simulink library "AuxEq_Lib"  (Simulink 8.0)
settings: Solver=ode45  SolverMode=SingleTasking  StartTime=0.0  StopTime=10.0  RelTol=1e-3
values from neighbouring files (symbols this model uses):
  TrimCondition =     [UAV_trimcondition.mat]
libraries: aerolibasang x3, Navigation_Lib x1, simulink x1
settings Model: Creator=Paul Freeman  LastModifiedBy=brtaylor

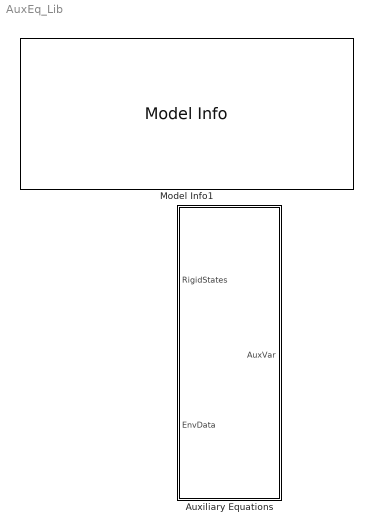
== system AuxEq_Lib ==
  Auxiliary Equations : Subsystem
  Model Info1 : simulink/Model-Wide Utilities/Model Info  InitialBlockCM=None  BlockCM=None  Frame=on  DisplayStringWithTags=|  HorizontalTextAlignment=Left  LeftAlignmentValue=0.02  SourceBlockDiagram=AuxEq_Lib  TagMaxNumber=20
      | MODEL INFORMATION
      | Auxiliary Equations Library
      | 
      | University of Minnesota
      | Aerospace Engineering and Mechanics
      | Copyright 2011 Regents of the University of Minnesota. All rights reserved.
      | 
      | == SVN Info ==
      | Last modified by %<LastModifiedBy> on %<LastModificationDate>

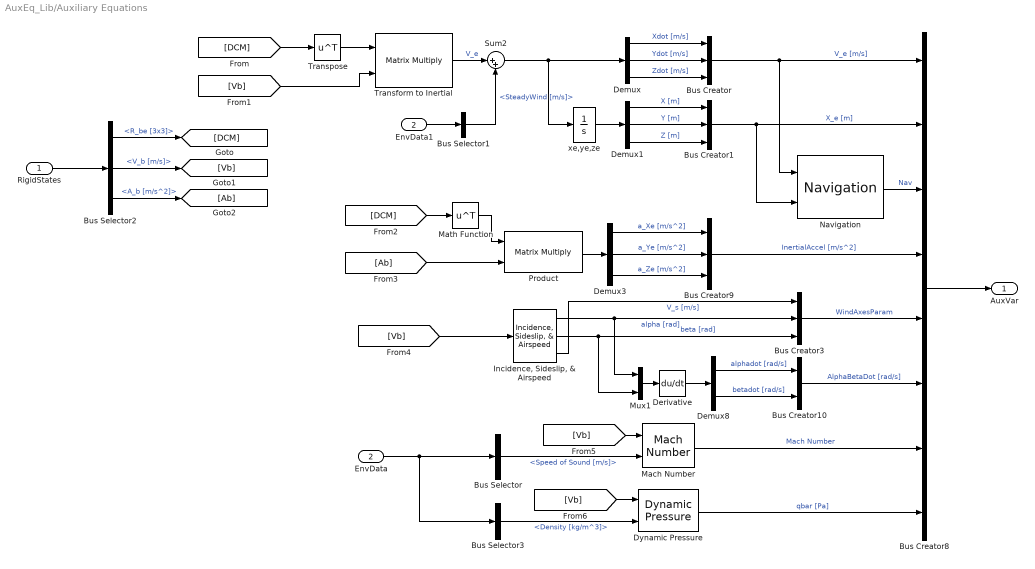
== system AuxEq_Lib/Auxiliary Equations ==
  RigidStates : Inport
  EnvData : Inport  Port=2
  Bus Creator{,1,3,9} (4 alike) : BusCreator  Inputs=3
  Bus Creator10 : BusCreator  Inputs=2
  Bus Creator8 : BusCreator  Inputs=8
  Bus Selector : BusSelector  OutputSignals=Speed of Sound [m/s]
  Bus Selector1 : BusSelector  OutputSignals=SteadyWind [m/s]
  Bus Selector2 : BusSelector  OutputSignals=R_be [3x3],V_b [m/s],A_b [m/s^2]
  Bus Selector3 : BusSelector  OutputSignals=Density [kg/m^3]
  Demux : Demux  Outputs=3
  Demux1 : Demux  Outputs=3
  Demux3 : Demux  Outputs=3
  Demux8 : Demux  Outputs=2
  Derivative : Derivative
  Dynamic Pressure : aerolibasang/Dynamic Pressure
  EnvData1 : InportShadow  Port=2
  "Incidence, Sideslip, & Airspeed" : aerolibasang/Incidence, Sideslip, & Airspeed
  Mach Number : aerolibasang/Mach Number
  Math Function : Math  Operator=transpose  SaturateOnIntegerOverflow=on
  Mux1 : Mux  Inputs=2
  Navigation : Navigation_Lib/Navigation  Description=|
      | This model produces the followng navigation data for the UAV flight:
      |                                                                     
      | * Geodetic Latitude                                                 
      | * Geodetic Longitude                                                
      | * Geodetic Altitude                                                 
      | * Altitude above Mean Sea Level                                     
      | * Gravitational acceleration vector
  Product : Product  Multiplication=Matrix(*)  RndMeth=Zero
  Sum2 : Sum  Inputs=|++
  Transform to Inertial : Product  Multiplication=Matrix(*)  RndMeth=Zero
  Transpose : Math  Operator=transpose  SaturateOnIntegerOverflow=on
  xe,ye,ze : Integrator  InitialCondition=TrimCondition.InertialIni
  AuxVar : Outport
  wires:
  RigidStates/1 -> Bus Selector2/1
  [Vb] -> Mach Number/1
  [Vb] -> "Incidence, Sideslip, & Airspeed"/1
  [DCM] -> Math Function/1
  [Ab] -> Product/2
  Mach Number/1 -> Bus Creator8/7  "Mach Number"
  Demux8/2 -> Bus Creator10/2  "betadot [rad/s]"
  Demux8/1 -> Bus Creator10/1  "alphadot [rad/s]"
  Bus Creator10/1 -> Bus Creator8/6  "AlphaBetaDot [rad/s]"
  Derivative/1 -> Demux8/1
  Mux1/1 -> Derivative/1
  "Incidence, Sideslip, & Airspeed"/3 -> Bus Creator3/1  "V_s [m/s]"
  "Incidence, Sideslip, & Airspeed"/2 -> Bus Creator3/3, Mux1/2  "beta [rad]"
  "Incidence, Sideslip, & Airspeed"/1 -> Bus Creator3/2, Mux1/1  "alpha [rad]"
  Bus Creator8/1 -> AuxVar/1
  Navigation/1 -> Bus Creator8/3  "Nav"
  Bus Creator9/1 -> Bus Creator8/4  "InertialAccel [m/s^2]"
  Demux3/2 -> Bus Creator9/2  "a_Ye [m/s^2]"
  Demux3/3 -> Bus Creator9/3  "a_Ze [m/s^2]"
  Demux3/1 -> Bus Creator9/1  "a_Xe [m/s^2]"
  Product/1 -> Demux3/1
  Math Function/1 -> Product/1
  Bus Selector/1 -> Mach Number/2  "<Speed of Sound [m/s]>"
  EnvData/1 -> Bus Selector3/1, Bus Selector/1
  Bus Creator3/1 -> Bus Creator8/5  "WindAxesParam"
  Demux1/3 -> Bus Creator1/3  "Z [m]"
  Demux1/2 -> Bus Creator1/2  "Y [m]"
  Demux1/1 -> Bus Creator1/1  "X [m]"
  Bus Creator1/1 -> Bus Creator8/2, Navigation/2  "X_e [m]"
  Demux/3 -> Bus Creator/3  "Zdot [m/s]"
  Demux/2 -> Bus Creator/2  "Ydot [m/s]"
  Demux/1 -> Bus Creator/1  "Xdot [m/s]"
  Bus Creator/1 -> Bus Creator8/1, Navigation/1  "V_e [m/s]"
  Transpose/1 -> Transform to Inertial/1
  [DCM] -> Transpose/1
  EnvData1/1 -> Bus Selector1/1
  Transform to Inertial/1 -> Sum2/1  "V_e"
  Bus Selector1/1 -> Sum2/2  "<SteadyWind [m/s]>"
  Sum2/1 -> Demux/1, xe,ye,ze/1
  xe,ye,ze/1 -> Demux1/1
  Bus Selector2/1 -> [DCM]  "<R_be [3x3]>"
  Bus Selector2/2 -> [Vb]  "<V_b [m/s]>"
  Bus Selector2/3 -> [Ab]  "<A_b [m/s^2]>"
  [Vb] -> Transform to Inertial/2
  [Vb] -> Dynamic Pressure/1
  Bus Selector3/1 -> Dynamic Pressure/2  "<Density [kg/m^3]>"
  Dynamic Pressure/1 -> Bus Creator8/8  "qbar [Pa]"
